simulink model "Drone_pos_ctrl"  (R2018b)
settings: Solver=ode2  StartTime=0.0  StopTime=T  FixedStep=Ts  RelTol=1e-3
values from neighbouring files (symbols this model uses):
  kd_d = 8    [drone_parameters.m]
  kd_phi = 8    [drone_parameters.m]
  kd_si = 8    [drone_parameters.m]
  kd_theta = 8    [drone_parameters.m]
  kd_z = 8    [drone_parameters.m]
  ki_d = 0.1    [drone_parameters.m]
  ki_phi = 0.5    [drone_parameters.m]
  ki_si = 0.5    [drone_parameters.m]
  ki_theta = 0.5    [drone_parameters.m]
  ki_z = 0.5    [drone_parameters.m]
  kp_d = 7    [drone_parameters.m]
  kp_phi = 7    [drone_parameters.m]
  kp_si = 7    [drone_parameters.m]
  kp_theta = 7    [drone_parameters.m]
  kp_z = 7    [drone_parameters.m]
  si_d = 1    [drone_parameters.m]
  T = 50    [drone_parameters.m]
  x_d = 20    [drone_parameters.m]
  y_d = 65    [drone_parameters.m]
  z_d = 50    [drone_parameters.m]
undefined symbols (not defined in the file or in its folder): droneOrientation, droneparam, dronePos
settings Model: Creator=saad  LastModifiedBy=root
settings SFSimCC: SimUseLocalCustomCode=off
settings RTWCC: RTWUseLocalCustomCode=off

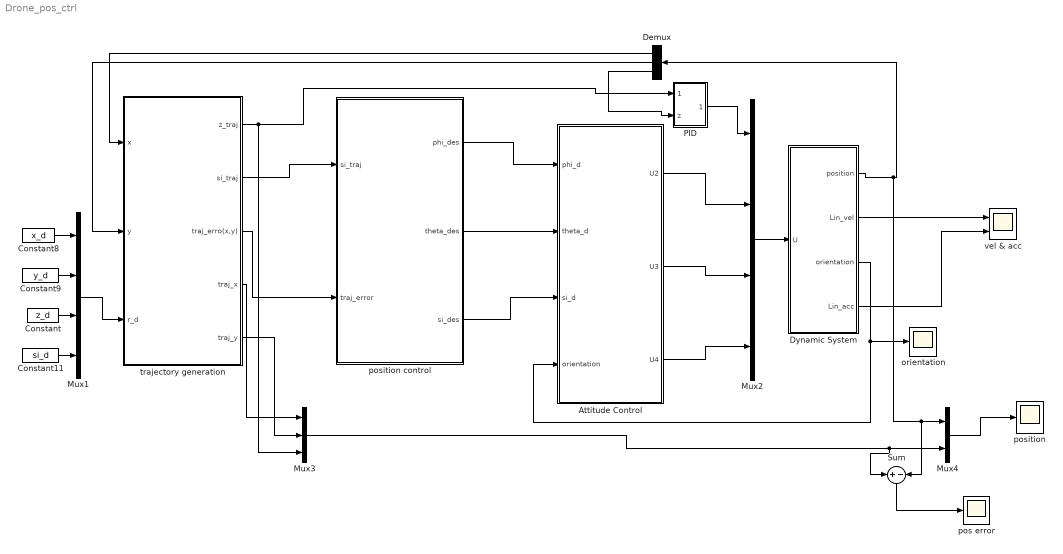
== system Drone_pos_ctrl ==
  Attitude Control : Subsystem
  Constant : Constant  Value=z_d
  Constant11 : Constant  Value=si_d
  Constant8 : Constant  Value=x_d
  Constant9 : Constant  Value=y_d
  Demux : Demux  Outputs=3
  "Dynamic System " : Subsystem
  Mux1 : Mux
  Mux2 : Mux
  Mux3 : Mux  Inputs=3
  Mux4 : Mux  Inputs=2
  PID : Subsystem
  Sum : Sum  Inputs=+-
  orientation : Scope
  "pos error " : Scope
  "position " : Scope
  position control : Subsystem
  trajectory generation : Subsystem
  vel & acc : Scope  NumInputPorts=2
  wires:
  PID/1(U1) -> Mux2/1
  "Dynamic System "/3(orientation) -> Attitude Control/4(orientation), orientation/1
  "Dynamic System "/1("position ") -> Sum/2, Mux4/1, Demux/1
  Demux/3 -> PID/2(z)
  Mux2/1 -> "Dynamic System "/1(U)
  Attitude Control/1(U2) -> Mux2/2
  Attitude Control/2(U3) -> Mux2/3
  Attitude Control/3(U4) -> Mux2/4
  position control/1(phi_des) -> Attitude Control/1(phi_d)
  position control/2(theta_des) -> Attitude Control/2(theta_d)
  position control/3(si_des) -> Attitude Control/3(si_d)
  Constant9/1 -> Mux1/2
  Constant8/1 -> Mux1/1
  Constant/1 -> Mux1/3
  Constant11/1 -> Mux1/4
  Demux/1 -> trajectory generation/1(x)
  Demux/2 -> trajectory generation/2(y)
  Mux1/1 -> trajectory generation/3(r_d)
  trajectory generation/1(z_traj) -> Mux3/3, PID/1(z_ref)
  trajectory generation/2(si_traj) -> position control/1(si_traj)
  trajectory generation/3(traj_erro(x,y)) -> position control/2(traj_error)
  trajectory generation/4(traj_x) -> Mux3/1
  trajectory generation/5(traj_y) -> Mux3/2
  Mux3/1 -> Sum/1, Mux4/2
  Mux4/1 -> "position "/1
  "Dynamic System "/4(Lin_acc) -> vel & acc/2
  "Dynamic System "/2(Lin_vel) -> vel & acc/1
  Sum/1 -> "pos error "/1

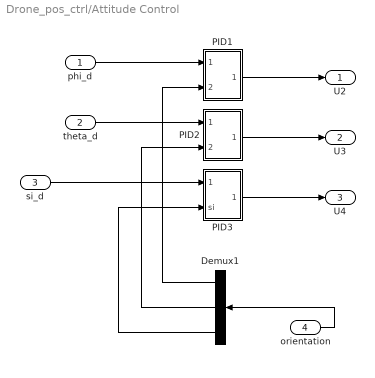
== system Drone_pos_ctrl/Attitude Control ==
  phi_d : Inport
  theta_d : Inport  Port=2
  si_d : Inport  Port=3
  orientation : Inport  Port=4
  Demux1 : Demux  Outputs=3
  PID1 : Subsystem
  PID2 : Subsystem
  PID3 : Subsystem
  U2 : Outport
  U3 : Outport  Port=2
  U4 : Outport  Port=3
  wires:
  PID3/1("U4 ") -> U4/1
  Demux1/1 -> PID1/2(phi)
  si_d/1 -> PID3/1(si_ref)
  PID2/1(U3) -> U3/1
  Demux1/3 -> PID3/2(si)
  Demux1/2 -> PID2/2(theta)
  PID1/1(U2) -> U2/1
  theta_d/1 -> PID2/1(theta_ref)
  phi_d/1 -> PID1/1(phi_ref)
  orientation/1 -> Demux1/1

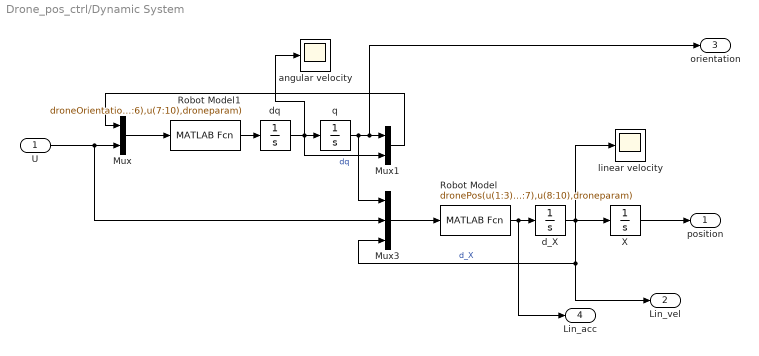
== system Drone_pos_ctrl/Dynamic System  ==
  U : Inport
  Mux : Mux  Inputs=2
  Mux1 : Mux  Inputs=2
  Mux3 : Mux  Inputs=3
  Robot Model : MATLABFcn  MATLABFcn=dronePos(u(1:3),u(4:7),u(8:10),droneparam)  OutputDimensions=3
  Robot Model1 : MATLABFcn  MATLABFcn=droneOrientation(u(1:3),u(4:6),u(7:10),droneparam)  OutputDimensions=3
  X : Integrator  InitialCondition=droneparam.X0
  angular velocity : Scope
  d_X : Integrator  InitialCondition=droneparam.X0
  dq : Integrator  InitialCondition=droneparam.q0
  "linear velocity " : Scope
  q : Integrator  InitialCondition=droneparam.q0
  "position " : Outport
  Lin_vel : Outport  Port=2
  orientation : Outport  Port=3
  Lin_acc : Outport  Port=4
  wires:
  Mux3/1 -> Robot Model/1
  q/1 -> Mux3/1, orientation/1, Mux1/1
  X/1 -> "position "/1
  U/1 -> Mux3/2, Mux/2
  Mux/1 -> Robot Model1/1
  Mux1/1 -> Mux/1
  dq/1 -> angular velocity/1, Mux1/2, q/1  "dq"
  Robot Model1/1 -> dq/1
  Robot Model/1 -> Lin_acc/1, d_X/1
  d_X/1 -> Lin_vel/1, Mux3/3, "linear velocity "/1, X/1  "d_X"

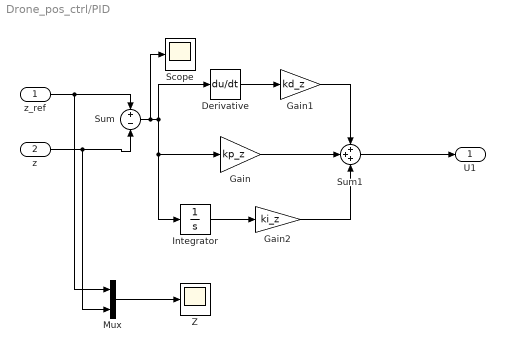
== system Drone_pos_ctrl/PID ==
  z_ref : Inport
  z : Inport  Port=2
  Derivative : Derivative
  Gain : Gain  Gain=kp_z
  Gain1 : Gain  Gain=kd_z
  Gain2 : Gain  Gain=ki_z
  Integrator : Integrator
  Mux : Mux  Inputs=2
  Scope : Scope
  Sum : Sum  Inputs=+-
  Sum1 : Sum  Inputs=+++
  Z : Scope
  U1 : Outport
  wires:
  Sum/1 -> Gain/1, Integrator/1, Derivative/1, Scope/1
  Integrator/1 -> Gain2/1
  Sum1/1 -> U1/1
  Gain/1 -> Sum1/2
  Gain2/1 -> Sum1/3
  Gain1/1 -> Sum1/1
  Derivative/1 -> Gain1/1
  z/1 -> Mux/2, Sum/2
  z_ref/1 -> Mux/1, Sum/1
  Mux/1 -> Z/1

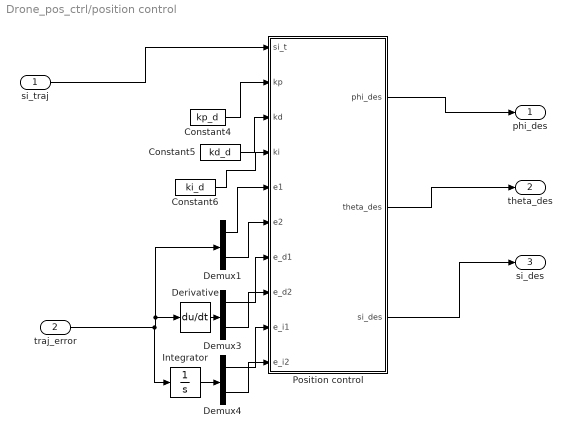
== system Drone_pos_ctrl/position control ==
  si_traj : Inport
  traj_error : Inport  Port=2
  Constant4 : Constant  Value=kp_d
  Constant5 : Constant  Value=kd_d
  Constant6 : Constant  Value=ki_d
  Demux1 : Demux  Outputs=2
  Demux3 : Demux  Outputs=2
  Demux4 : Demux  Outputs=2
  Derivative : Derivative
  Integrator : Integrator
  Position control : MATLAB Function  TreatAsAtomicUnit=on
  phi_des : Outport
  theta_des : Outport  Port=2
  si_des : Outport  Port=3
  wires:
  si_traj/1 -> Position control/1(si_t)
  Demux3/2 -> Position control/8(e_d2)
  traj_error/1 -> Integrator/1, Demux1/1, Derivative/1
  Demux4/2 -> Position control/10(e_i2)
  Demux1/2 -> Position control/6(e2)
  Demux1/1 -> Position control/5(e1)
  Constant6/1 -> Position control/4(ki)
  Constant4/1 -> Position control/2(kp)
  Position control/2(theta_des) -> theta_des/1
  Position control/3(si_des) -> si_des/1
  Constant5/1 -> Position control/3(kd)
  Position control/1(phi_des) -> phi_des/1
  Integrator/1 -> Demux4/1
  Demux4/1 -> Position control/9(e_i1)
  Derivative/1 -> Demux3/1
  Demux3/1 -> Position control/7(e_d1)

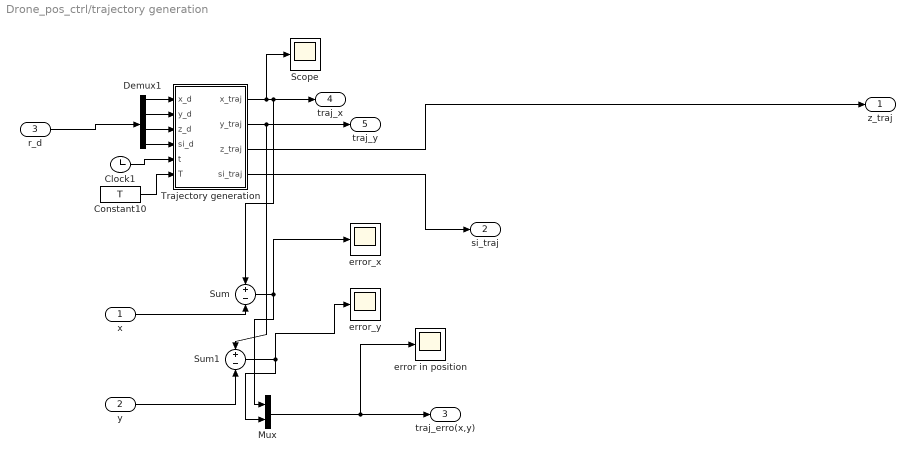
== system Drone_pos_ctrl/trajectory generation ==
  x : Inport
  y : Inport  Port=2
  r_d : Inport  Port=3
  Clock1 : Clock
  Constant10 : Constant  Value=T
  Demux1 : Demux
  Mux : Mux  Inputs=2
  Scope : Scope
  Sum : Sum  Inputs=+-
  Sum1 : Sum  Inputs=+-
  Trajectory generation : MATLAB Function  TreatAsAtomicUnit=on
  error in position : Scope
  error_x : Scope
  error_y : Scope
  z_traj : Outport
  si_traj : Outport  Port=2
  traj_erro(x,y) : Outport  Port=3
  traj_x : Outport  Port=4
  traj_y : Outport  Port=5
  wires:
  Clock1/1 -> Trajectory generation/5(t)
  Sum1/1 -> Mux/2, error_y/1
  Sum/1 -> Mux/1, error_x/1
  x/1 -> Sum/2
  y/1 -> Sum1/2
  Trajectory generation/1(x_traj) -> Scope/1, traj_x/1, Sum/1
  Mux/1 -> error in position/1, traj_erro(x,y)/1
  Trajectory generation/4(si_traj) -> si_traj/1
  Demux1/2 -> Trajectory generation/2(y_d)
  Trajectory generation/2(y_traj) -> traj_y/1, Sum1/1
  Demux1/1 -> Trajectory generation/1(x_d)
  Demux1/4 -> Trajectory generation/4(si_d)
  r_d/1 -> Demux1/1
  Constant10/1 -> Trajectory generation/6(T)
  Trajectory generation/3(z_traj) -> z_traj/1
  Demux1/3 -> Trajectory generation/3(z_d)

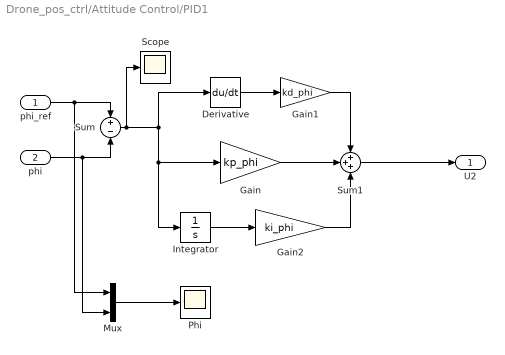
== system Drone_pos_ctrl/Attitude Control/PID1 ==
  phi_ref : Inport
  phi : Inport  Port=2
  Derivative : Derivative
  Gain : Gain  Gain=kp_phi
  Gain1 : Gain  Gain=kd_phi
  Gain2 : Gain  Gain=ki_phi
  Integrator : Integrator
  Mux : Mux  Inputs=2
  Phi : Scope
  Scope : Scope
  Sum : Sum  Inputs=+-
  Sum1 : Sum  Inputs=+++
  U2 : Outport
  wires:
  Derivative/1 -> Gain1/1
  Gain1/1 -> Sum1/1
  phi/1 -> Mux/2, Sum/2
  Gain2/1 -> Sum1/3
  Gain/1 -> Sum1/2
  Sum1/1 -> U2/1
  Integrator/1 -> Gain2/1
  Sum/1 -> Scope/1, Derivative/1, Integrator/1, Gain/1
  phi_ref/1 -> Mux/1, Sum/1
  Mux/1 -> Phi/1

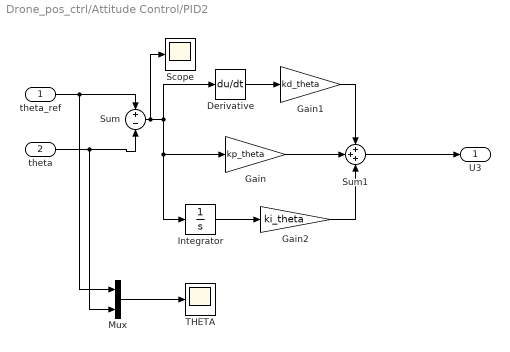
== system Drone_pos_ctrl/Attitude Control/PID2 ==
  theta_ref : Inport
  theta : Inport  Port=2
  Derivative : Derivative
  Gain : Gain  Gain=kp_theta
  Gain1 : Gain  Gain=kd_theta
  Gain2 : Gain  Gain=ki_theta
  Integrator : Integrator
  Mux : Mux  Inputs=2
  Scope : Scope
  Sum : Sum  Inputs=+-
  Sum1 : Sum  Inputs=+++
  "THETA " : Scope
  U3 : Outport
  wires:
  Sum/1 -> Gain/1, Integrator/1, Derivative/1, Scope/1
  Integrator/1 -> Gain2/1
  Sum1/1 -> U3/1
  Gain/1 -> Sum1/2
  Gain2/1 -> Sum1/3
  Gain1/1 -> Sum1/1
  Derivative/1 -> Gain1/1
  theta/1 -> Mux/2, Sum/2
  theta_ref/1 -> Mux/1, Sum/1
  Mux/1 -> "THETA "/1

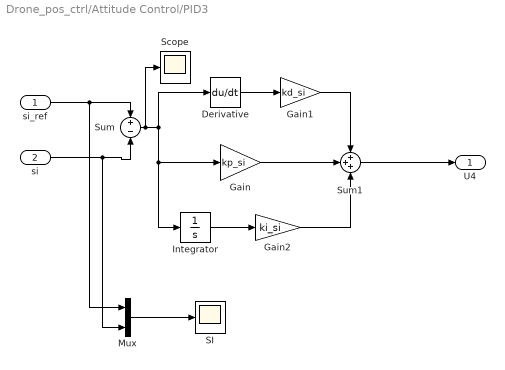
== system Drone_pos_ctrl/Attitude Control/PID3 ==
  si_ref : Inport
  si : Inport  Port=2
  Derivative : Derivative
  Gain : Gain  Gain=kp_si
  Gain1 : Gain  Gain=kd_si
  Gain2 : Gain  Gain=ki_si
  Integrator : Integrator
  Mux : Mux  Inputs=2
  SI : Scope
  Scope : Scope
  Sum : Sum  Inputs=+-
  Sum1 : Sum  Inputs=+++
  "U4 " : Outport
  wires:
  Derivative/1 -> Gain1/1
  Gain1/1 -> Sum1/1
  Gain2/1 -> Sum1/3
  Gain/1 -> Sum1/2
  Sum1/1 -> "U4 "/1
  Integrator/1 -> Gain2/1
  Sum/1 -> Integrator/1, Gain/1, Derivative/1, Scope/1
  si/1 -> Mux/2, Sum/2
  si_ref/1 -> Mux/1, Sum/1
  Mux/1 -> SI/1

== matlab function Drone_pos_ctrl/trajectory generation/Trajectory generation ==
  data: x_d input; x_traj output; y_d input; z_d input; si_d input; t input; T input; y_traj output; z_traj output; si_traj output
function [x_traj,y_traj,z_traj,si_traj] = fcn(x_d,y_d,z_d,si_d,t,T)
  % min velocity trajectory
    x_traj = x_d*t^2/T^2;
   y_traj = y_d*t^2/T^2;
    si_traj = si_d*t^2/T^2;
    z_traj = z_d*t^2/T^2;
    
     % min acc trajectory
    %x_traj = x_d*t^3/T^3;
    %y_traj = y_d*t^3/T^3;
    %si_traj = si_d*t^3/T^3;
    %z_traj = z_d*t^3/T^3;
    
    %min distance traj
    %x_traj = x_d*t/T;
    %y_traj = y_d*t/T;
    %si_traj = si_d*t/T;
   % z_traj = z_d;
   
end

== matlab function Drone_pos_ctrl/position control/Position control ==
  data: si_t input; kp input; kd input; ki input; phi_des output; e1 input; theta_des output; e2 input; e_d1 input; si_des output; e_d2 input; e_i1 input; e_i2 input
function [phi_des,theta_des,si_des] = fcn(si_t,kp,kd,ki,e1,e2,e_d1,e_d2,e_i1,e_i2)
        e = [e1 e2];
        e_d = [e_d1 e_d2];
        e_i = [e_i1 e_i2];
   
    
    ddr_des = kd*e_d + kp*e + ki*e_i;
    
    phi_des = (ddr_des(1)*sin(si_t) - ddr_des(2)*cos(si_t))/9.8;
    
    theta_des = (ddr_des(1)*cos(si_t) + ddr_des(2)*sin(si_t))/9.8;
    
    si_des = si_t;
end
